simulink model "Model_2"  (R2020b)
settings: Solver=VariableStepAuto  StartTime=0.0  StopTime=100  RelTol=1e-3
settings Model: Creator=Akarsh  LastModifiedBy=Akarsh

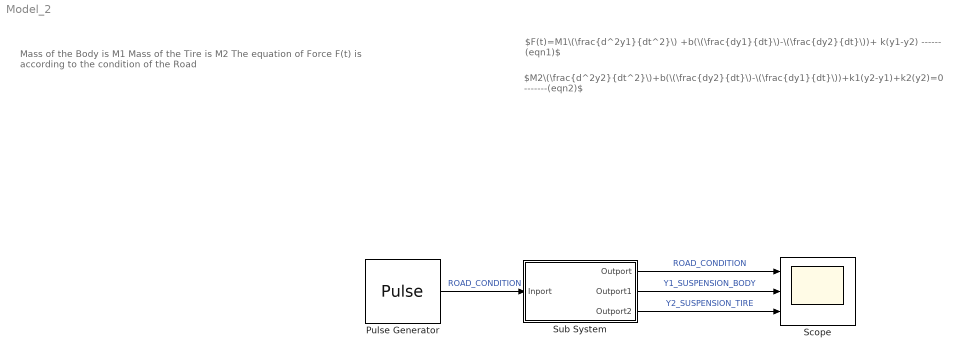
== system Model_2 ==
  note: Mass of the Body is M1
      | Mass of the Tire is M2
      | The equation of Force F(t) is according to the condition of the Road
  note: $F(t)=M1\(\frac{d^2y1}{dt^2}\) +b(\(\frac{dy1}{dt}\)-\(\frac{dy2}{dt}\))+ k(y1-y2) ------ (eqn1)$
  note: $M2\(\frac{d^2y2}{dt^2}\)+b(\(\frac{dy2}{dt}\)-\(\frac{dy1}{dt}\))+k1(y2-y1)+k2(y2)=0 -------(eqn2)$
  " Sub System" : Subsystem
  Pulse Generator : DiscretePulseGenerator  PulseType=Time based  Period=20  PulseWidth=5
  Scope : Scope  NumInputPorts=3
  wires:
  " Sub System"/2(Outport1) -> Scope/2  "Y1_SUSPENSION_BODY"
  " Sub System"/1(Outport) -> Scope/1  "ROAD_CONDITION"
  " Sub System"/3(Outport2) -> Scope/3  "Y2_SUSPENSION_TIRE"
  Pulse Generator/1 -> " Sub System"/1(Inport)  "ROAD_CONDITION"

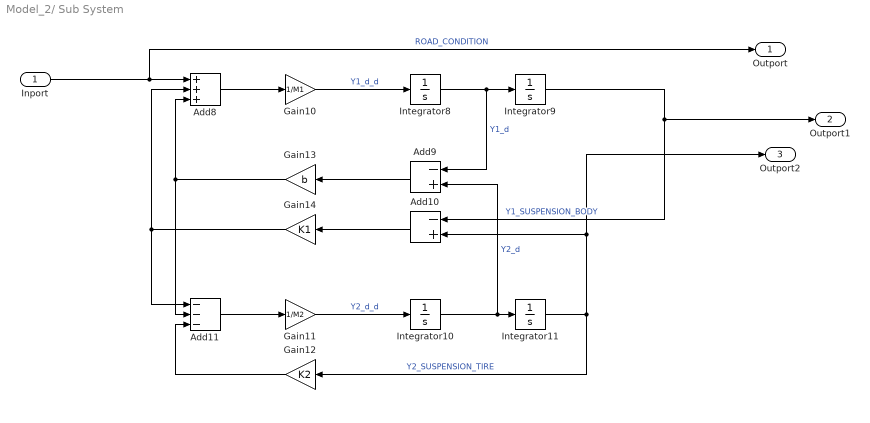
== system Model_2/ Sub System ==
  Inport : Inport
  Add10 : Sum  Inputs=-+
  Add11 : Sum  Inputs=---
  Add8 : Sum  Inputs=+++
  Add9 : Sum  Inputs=-+
  Gain10 : Gain  Gain=1/M1  mask{M1=0.001}
  Gain11 : Gain  Gain=1/M2  mask{M2=0.03}
  Gain12 : Gain  Gain=K2  mask{K2=100}
  Gain13 : Gain  Gain=b  mask{b=0.1}
  Gain14 : Gain  Gain=K1  mask{K1=0.75}
  Integrator{8..11} (4 alike) : Integrator
  Outport : Outport
  Outport1 : Outport  Port=2
  Outport2 : Outport  Port=3
  wires:
  Integrator9/1 -> Outport1/1, Add10/1  "Y1_SUSPENSION_BODY"
  Integrator8/1 -> Integrator9/1, Add9/1  "Y1_d"
  Gain13/1 -> Add11/2, Add8/3
  Add8/1 -> Gain10/1
  Add9/1 -> Gain13/1
  Inport/1 -> Outport/1, Add8/1  "ROAD_CONDITION"
  Gain10/1 -> Integrator8/1  "Y1_d_d"
  Integrator10/1 -> Add9/2, Integrator11/1  "Y2_d"
  Add10/1 -> Gain14/1
  Gain11/1 -> Integrator10/1  "Y2_d_d"
  Integrator11/1 -> Outport2/1, Add10/2, Gain12/1  "Y2_SUSPENSION_TIRE"
  Gain14/1 -> Add11/1, Add8/2
  Add11/1 -> Gain11/1
  Gain12/1 -> Add11/3
